simulink model "FlightGearInterface"  (R2024b)
settings: Solver=VariableStepAuto  StartTime=0.0  StopTime=10.0  RelTol=1e-3
libraries: aerolibfltsims x2
settings Model: Creator=the-main  LastModifiedBy=the-main

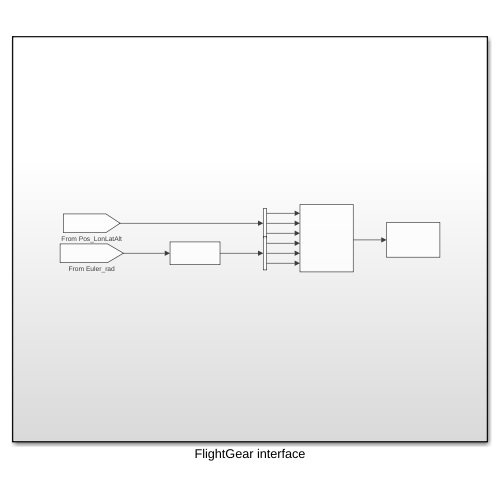
[thumbnail: Simulink's stored preview of the top-level diagram]
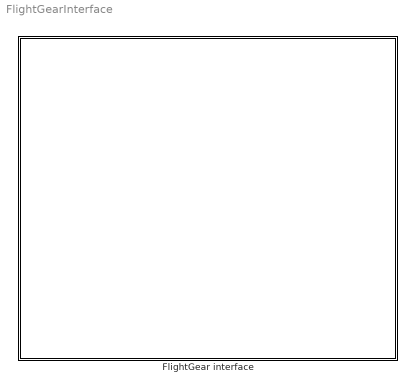
== system FlightGearInterface ==
  FlightGear interface : Subsystem

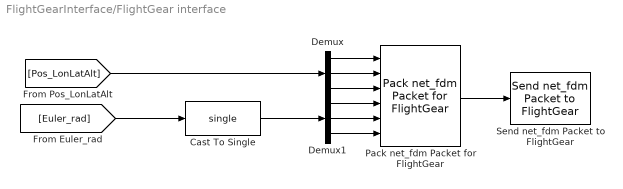
== system FlightGearInterface/FlightGear interface ==
  Cast To Single : DataTypeConversion  OutDataTypeStr=single  SaturateOnIntegerOverflow=off  RndMeth=Floor
  Demux : Demux  Outputs=3
  Demux1 : Demux  Outputs=3
  Pack net_fdm Packet for FlightGear : aerolibfltsims/Pack net_fdm Packet for FlightGear  FlightGearVersion=v2019.1  ShowPositionAttitudeInputs=on  ShowVelocityAccelerationInputs=off  ShowControlSurfacePositionInputs=off  ShowEngineFuelInputs=off  ShowLandingGearInputs=off  ShowEnvironmentInputs=off  SampleTime=1/30  packetVersion=24
  Send net_fdm Packet to FlightGear : aerolibfltsims/Send net_fdm Packet to FlightGear  DestinationIpAddress=127.0.0.1  DestinationPort=5502  LocalIpPort=-1  varLen=off  SampleTime=1/30
  wires:
  Pack net_fdm Packet for FlightGear/1 -> Send net_fdm Packet to FlightGear/1
  [Pos_LonLatAlt] -> Demux/1
  Demux/1 -> Pack net_fdm Packet for FlightGear/1
  Demux/2 -> Pack net_fdm Packet for FlightGear/2
  Demux/3 -> Pack net_fdm Packet for FlightGear/3
  [Euler_rad] -> Cast To Single/1
  Cast To Single/1 -> Demux1/1
  Demux1/1 -> Pack net_fdm Packet for FlightGear/4
  Demux1/2 -> Pack net_fdm Packet for FlightGear/5
  Demux1/3 -> Pack net_fdm Packet for FlightGear/6
